simulink model "car_model"  (R2022b)
settings: Solver=VariableStepAuto  StartTime=0.0  StopTime=30  RelTol=1e-3
values from neighbouring files (symbols this model uses):
  X = Chassis_Signals.InertFrm.Cg.Disp.X.Data(:)    [Simulation_Data_Parse.m]    (also in Vehicle_Sim_Parse.m)
  Y = Chassis_Signals.InertFrm.Cg.Disp.Y.Data(:)    [Simulation_Data_Parse.m]    (also in Vehicle_Sim_Parse.m)
undefined symbols (not defined in the file or in its folder): ABS_MAX_TORQUE, ABS_MAX_TRQ_CMD, ABS_MIN_TORQUE, acc_IC, ACCELERATION_MAX, ActSuspDutyCycle, Aeq_left, Aeq_right, alpha_error, ang_acc_hystersesis, ang_IC, ang_vel_IC, area_air, axb, battery_current_IC, BATTERY_CURRENT_MAX, BATTERY_CURRENT_MIN, battery_FT_IC, battery_T_IC, BATTERY_TEMPERATURE_MAX, BATTERY_TEMPERATURE_MIN, battery_voltage_IC, BATTERY_VOLTAGE_MAX, BATTERY_VOLTAGE_MIN, Brake_Pressure_IC, ccl_IC, CENTER_STEER_ANGLE_MAX, covA, covarience_matrix_IC, covG, covM, covP, covV, cy_sweep, dB, dcl_IC, DCL_MAX, DCL_MIN, deadband_angle, dIndex, DiscIntNeverNeededParam, disk_abore, driver_t, dt_OFF, dt_ON, dTx, dx, dZ, F0z, forward_look_straight, forward_look_turn, fusion_t, fusion_t_sim, Fz_IC, Fz_sweep, g, gearbox_efficiency, gps_counter_IC, gps_ratio, gr ... (+105)
libraries: fl_lib x62, nesl_utility x16, vehdynlibtire x10, vehdynlibsuspension x8, simulink x5, autolibutils x5, sharedtransform x5, EngineCoolingComponents_lib x4, slpidlib x3, SimscapeFluids_lib x3, dspstat3 x2, shared6dof x2
(part 3 of 10)

== system car_model/Vehicle Model/Electronics/Cooling Sensors ==
  Analog Signals : Inport
  Bus Creator9 : BusCreator  Inputs=5
  Bus Selector : BusSelector  OutputSignals=trn.motor_temperature,trn.mc_temp,trn.motor_fluid_temperature,trn.battery_temperature,trn.battery_fluid_temperature
  Delay1 : Delay  InitialCondition=[1 1; 1 1; 1 1; 1 1].*motor_T_IC
  Delay11 : Delay  InitialCondition=[1 1; 1 1; 1 1; 1 1].*motor_T_IC
  Delay12 : Delay  InitialCondition=[1 1; 1 1].*motor_FT_IC
  Delay13 : Delay  InitialCondition=[1 1].*battery_T_IC
  Delay14 : Delay  InitialCondition=[1 1].*battery_FT_IC
  Rate Transition1 : RateTransition  InitialCondition=[1 1].*motor_FT_IC  OutPortSampleTime=0
  Rate Transition2 : RateTransition  OutPortSampleTime=0
  Rate Transition3 : RateTransition  OutPortSampleTime=0
  Saturation10 : Saturate  UpperLimit=MOTOR_TEMPERATURE_MAX  LowerLimit=MOTOR_TEMPERATURE_MIN
  Saturation11 : Saturate  UpperLimit=BATTERY_TEMPERATURE_MAX  LowerLimit=BATTERY_TEMPERATURE_MIN
  Saturation12 : Saturate  UpperLimit=BATTERY_TEMPERATURE_MAX  LowerLimit=BATTERY_TEMPERATURE_MIN
  Saturation18 : Saturate  UpperLimit=MOTOR_TEMPERATURE_MAX  LowerLimit=MOTOR_TEMPERATURE_MIN
  Saturation21 : Saturate  UpperLimit=MOTOR_TEMPERATURE_MAX  LowerLimit=MOTOR_TEMPERATURE_MIN
  Zero-Order Hold{1,11..14} (5 alike) : ZeroOrderHold  SampleTime=sensor_t
  Cooling Sensors : Outport
  wires:
  Delay1/1 -> Saturation21/1
  Saturation21/1 -> Bus Creator9/2  "mc_T"
  Bus Selector/2 -> Zero-Order Hold1/1  "<mc_temp>"
  Zero-Order Hold1/1 -> Delay1/1
  Delay14/1 -> Saturation12/1
  Delay11/1 -> Saturation18/1
  Delay12/1 -> Saturation10/1
  Saturation12/1 -> Bus Creator9/5  "batt_FT"
  Zero-Order Hold12/1 -> Delay12/1
  Zero-Order Hold14/1 -> Delay14/1
  Bus Selector/4 -> Rate Transition2/1  "<battery_temperature>"
  Zero-Order Hold11/1 -> Delay11/1
  Saturation18/1 -> Bus Creator9/1  "motor_T"
  Zero-Order Hold13/1 -> Delay13/1
  Bus Selector/3 -> Rate Transition1/1  "<motor_fluid_temperature>"
  Saturation11/1 -> Bus Creator9/4  "batt_T"
  Saturation10/1 -> Bus Creator9/3  "motor_FT"
  Delay13/1 -> Saturation11/1
  Bus Selector/1 -> Zero-Order Hold11/1  "<motor_temperature>"
  Bus Selector/5 -> Rate Transition3/1  "<battery_fluid_temperature>"
  Bus Creator9/1 -> Cooling Sensors/1
  Rate Transition1/1 -> Zero-Order Hold12/1  "motor_fluid_temperature"
  Rate Transition2/1 -> Zero-Order Hold13/1  "battery_temperature"
  Rate Transition3/1 -> Zero-Order Hold14/1  "battery_fluid_temperature"
  Analog Signals/1 -> Bus Selector/1

== system car_model/Vehicle Model/Electronics/Corner Dynamics Sensors ==
  Analog Signals : Inport
  Bus Creator10 : BusCreator  Inputs=4
  Bus Selector : BusSelector  OutputSignals=whl.TireFrame.Omega,sus.Sus.steering_angle,sus.Sus.shock_length,whl.TireFrame.GndFz
  Delay15 : Delay  InitialCondition=ones(1, 4, 2).*omega_IC
  Delay16 : Delay  InitialCondition=[1 1].*theta_IC
  Delay17 : Delay  InitialCondition=[1 1; 1 1; 1 1; 1 1].*shock_length_IC
  Delay18 : Delay  InitialCondition=[1 1; 1 1; 1 1; 1 1].*Fz_IC
  Saturation15 : Saturate  UpperLimit=SHOCK_LENGTH_MAX  LowerLimit=SHOCK_LENGTH_MIN
  Saturation16 : Saturate  UpperLimit=OMEGA_MAX  LowerLimit=OMEGA_MIN
  Saturation17 : Saturate  UpperLimit=1200  LowerLimit=200
  Saturation3 : Saturate  UpperLimit=CENTER_STEER_ANGLE_MAX  LowerLimit=-CENTER_STEER_ANGLE_MAX
  Transpose : Math  Operator=transpose
  Zero-Order Hold{15..18} (4 alike) : ZeroOrderHold  SampleTime=sensor_t
  Corner Dynamics Sensors : Outport
  wires:
  Transpose/1 -> Zero-Order Hold15/1  "omega"
  Bus Selector/1 -> Transpose/1  "<Omega>"
  Zero-Order Hold18/1 -> Delay18/1
  Delay18/1 -> Saturation17/1
  Zero-Order Hold15/1 -> Delay15/1
  Zero-Order Hold16/1 -> Delay16/1
  Saturation17/1 -> Bus Creator10/4  "FZ"
  Saturation3/1 -> Bus Creator10/2  "theta"
  Bus Selector/3 -> Zero-Order Hold17/1  "<shock_length>"
  Saturation15/1 -> Bus Creator10/3  "shock_L"
  Saturation16/1 -> Bus Creator10/1  "omega"
  Bus Selector/4 -> Zero-Order Hold18/1  "<GndFz>"
  Delay16/1 -> Saturation3/1
  Bus Selector/2 -> Zero-Order Hold16/1  "<steering_angle>"
  Delay17/1 -> Saturation15/1
  Delay15/1 -> Saturation16/1
  Zero-Order Hold17/1 -> Delay17/1
  Bus Creator10/1 -> Corner Dynamics Sensors/1
  Analog Signals/1 -> Bus Selector/1

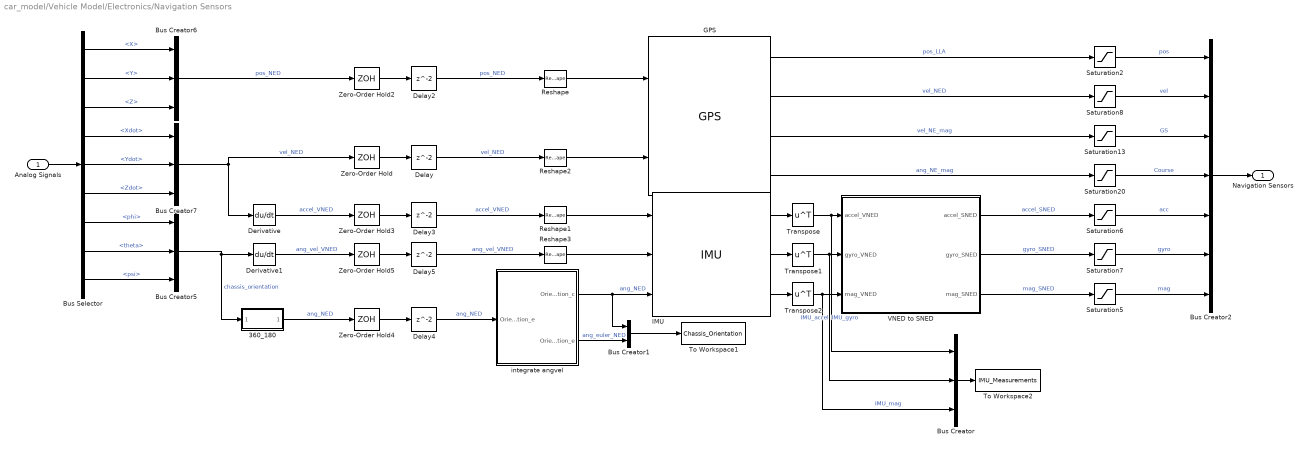
== system car_model/Vehicle Model/Electronics/Navigation Sensors ==
  Analog Signals : Inport
  360_180 : Subsystem
  Bus Creator : BusCreator  Inputs=IMU_accel,IMU_gyro,IMU_mag
  Bus Creator1 : BusCreator  Inputs=2
  Bus Creator2 : BusCreator  Inputs=7
  Bus Creator5 : BusCreator  Inputs=phi,theta,psi
  Bus Creator6 : BusCreator  Inputs=X,Y,Z
  Bus Creator7 : BusCreator  Inputs=Xdot,Ydot,Zdot
  Bus Selector : BusSelector  OutputSignals=veh.InertFrm.Cg.Disp.X,veh.InertFrm.Cg.Disp.Y,veh.InertFrm.Cg.Disp.Z,veh.InertFrm.Cg.Vel.Xdot,veh.InertFrm.Cg.Vel.Ydot,veh.InertFrm.Cg.Vel.Zdot,veh.InertFrm.Cg.Ang.phi,veh.InertFrm.Cg.Ang.theta,veh.InertFrm.Cg.Ang.psi
  Delay : Delay  InitialCondition=([1;1]*vel_IC)'
  Delay2 : Delay  InitialCondition=[1 1; 1 1; 1 1].*pos_IC
  Delay3 : Delay  InitialCondition=[1 1; 1 1; 1 1].*acc_IC
  Delay4 : Delay  InitialCondition=[1 1; 1 1; 1 1].*ang_IC
  Delay5 : Delay  InitialCondition=[1 1; 1 1; 1 1].*ang_vel_IC
  Derivative : Derivative
  Derivative1 : Derivative
  GPS : sensorgpslib/GPS  DispRefFrame=NED  PositionInputFormat=Local  ReferenceLocation=location_lla_IC  HorizontalPositionAccuracy=GPS_Z_ACCURACY  VerticalPositionAccuracy=GPS_XY_ACCURACY  VelocityAccuracy=GPS_V_ACCURACY  DecayFactor=GPS_NOISE_FACTOR  SeedDouble=r_GPS  SimulateUsing=Interpreted execution
      settings: LibrarySourceBlock=mspsensorlib/GPS
  IMU : mspsensorlib/IMU  DispRefFrame=NED  Temperature=25  MagneticFieldNED=mag_field_IC  MagneticFieldENU=[ -2.4169, 27.5550, 16.0849 ]  SeedDouble=r_IMU  SimulateUsing=Interpreted execution  AccelParamsMeasurementRange=ACC_MAX  AccelParamsResolution=ACC_RES  AccelParamsConstantBias=ACC_BIAS  AccelParamsAxesMisalignment=ACC_SKEW  AccelParamsNoiseDensity=ACC_VEL_WALK  AccelParamsBiasInstability=ACC_BIAS_INSTABILITY  AccelParamsRandomWalk=ACC_WALK  AccelParamsTemperatureBias=ACC_T_BIAS  AccelParamsTemperatureScaleFactor=ACC_T_SCALE  GyroParamsMeasurementRange=GYR_MAX  GyroParamsResolution=GYR_RES  GyroParamsConstantBias=GYR_BIAS  GyroParamsAxesMisalignment=GYR_SKEW  GyroParamsAccelerationBias=GYR_ACC_BIAS  GyroParamsNoiseDensity=GYR_ANG_WALK  GyroParamsBiasInstability=GYR_BIAS_INSTABILITY  GyroParamsRandomWalk=GYR_WALK  GyroParamsTemperatureBias=GYR_T_BIAS  GyroParamsTemperatureScaleFactor=GYR_T_SCALE  MagParamsMeasurementRange=MAG_MAX  MagParamsResolution=MAG_RES  MagParamsConstantBias=MAG_BIAS  MagParamsAxesMisalignment=MAG_SKEW  MagParamsNoiseDensity=MAG_WHITE  MagParamsBiasInstability=MAG_BIAS_INSTABILITY  MagParamsRandomWalk=MAG_WALK  MagParamsTemperatureBias=MAG_T_BIAS  MagParamsTemperatureScaleFactor=MAG_T_SCALE
  Reshape{,1..3} (4 alike) : Reshape  OutputDimensionality=Row vector (2-D)
  Saturation13 : Saturate  UpperLimit=VELOCITY_MAX  LowerLimit=-VELOCITY_MAX
  Saturation2 : Saturate  UpperLimit=inf  LowerLimit=-inf
  Saturation20 : Saturate  UpperLimit=ORIENTATION_MAX  LowerLimit=-ORIENTATION_MAX
  Saturation5 : Saturate  UpperLimit=MAG_MAX  LowerLimit=-MAG_MAX
  Saturation6 : Saturate  UpperLimit=ACCELERATION_MAX  LowerLimit=-ACCELERATION_MAX
  Saturation7 : Saturate  UpperLimit=YAW_MAX  LowerLimit=-YAW_MAX
  Saturation8 : Saturate  UpperLimit=VELOCITY_MAX  LowerLimit=-VELOCITY_MAX
  To Workspace1 : ToWorkspace  VariableName=Chassis_Orientation  SaveFormat=Timeseries  SampleTime=-1
  To Workspace2 : ToWorkspace  VariableName=IMU_Measurements  SaveFormat=Timeseries  SampleTime=-1
  Transpose : Math  Operator=transpose
  Transpose1 : Math  Operator=transpose
  Transpose2 : Math  Operator=transpose
  VNED to SNED : MATLAB Function  TreatAsAtomicUnit=on
  Zero-Order Hold{,2..5} (5 alike) : ZeroOrderHold  SampleTime=sensor_t
  integrate angvel : MATLAB Function  TreatAsAtomicUnit=on
  Navigation Sensors : Outport
  wires:
  Delay5/1 -> Reshape3/1  "ang_vel_VNED"
  Delay/1 -> Reshape2/1  "vel_NED"
  Delay3/1 -> Reshape1/1  "accel_VNED"
  Delay2/1 -> Reshape/1  "pos_NED"
  integrate angvel/1(Orientation_c) -> Bus Creator1/1, IMU/3  "ang_NED"
  GPS/4 -> Saturation20/1  "ang_NE_mag"
  GPS/3 -> Saturation13/1  "vel_NE_mag"
  GPS/2 -> Saturation8/1  "vel_NED"
  GPS/1 -> Saturation2/1  "pos_LLA"
  VNED to SNED/2(gyro_SNED) -> Saturation7/1  "gyro_SNED"
  VNED to SNED/1(accel_SNED) -> Saturation6/1  "accel_SNED"
  VNED to SNED/3(mag_SNED) -> Saturation5/1  "mag_SNED"
  Delay4/1 -> integrate angvel/1("Orientation_e ")  "ang_NED"
  Transpose2/1 -> Bus Creator/3, VNED to SNED/3(mag_VNED)  "IMU_mag"
  Transpose1/1 -> Bus Creator/2, VNED to SNED/2(gyro_VNED)  "IMU_gyro"
  Transpose/1 -> Bus Creator/1, VNED to SNED/1(accel_VNED)  "IMU_accel"
  IMU/3 -> Transpose2/1
  IMU/1 -> Transpose/1
  IMU/2 -> Transpose1/1
  Bus Creator/1 -> To Workspace2/1
  Bus Creator1/1 -> To Workspace1/1
  integrate angvel/2(Orientation_e) -> Bus Creator1/2  "ang_euler_NED"
  Zero-Order Hold/1 -> Delay/1
  Bus Creator7/1 -> Zero-Order Hold/1, Derivative/1  "vel_NED"
  Zero-Order Hold2/1 -> Delay2/1
  Bus Creator6/1 -> Zero-Order Hold2/1  "pos_NED"
  Zero-Order Hold3/1 -> Delay3/1
  Derivative/1 -> Zero-Order Hold3/1  "accel_VNED"
  Zero-Order Hold5/1 -> Delay5/1
  Derivative1/1 -> Zero-Order Hold5/1  "ang_vel_VNED"
  Zero-Order Hold4/1 -> Delay4/1
  360_180/1(psi_rev) -> Zero-Order Hold4/1  "ang_NED"
  Saturation2/1 -> Bus Creator2/1  "pos"
  Saturation13/1 -> Bus Creator2/3  "GS"
  Saturation6/1 -> Bus Creator2/5  "acc"
  Saturation20/1 -> Bus Creator2/4  "Course"
  Saturation5/1 -> Bus Creator2/7  "mag"
  Saturation8/1 -> Bus Creator2/2  "vel"
  Saturation7/1 -> Bus Creator2/6  "gyro"
  Bus Creator2/1 -> Navigation Sensors/1
  Bus Selector/1 -> Bus Creator6/1  "<X>"
  Bus Selector/8 -> Bus Creator5/2  "<theta>"
  Bus Selector/2 -> Bus Creator6/2  "<Y>"
  Bus Selector/6 -> Bus Creator7/3  "<Zdot>"
  Bus Selector/5 -> Bus Creator7/2  "<Ydot>"
  Bus Selector/4 -> Bus Creator7/1  "<Xdot>"
  Bus Selector/7 -> Bus Creator5/1  "<phi>"
  Bus Creator5/1 -> 360_180/1(<psi>), Derivative1/1  "chassis_orientation"
  Bus Selector/3 -> Bus Creator6/3  "<Z>"
  Bus Selector/9 -> Bus Creator5/3  "<psi>"
  Analog Signals/1 -> Bus Selector/1
  Reshape/1 -> GPS/1
  Reshape1/1 -> IMU/1
  Reshape2/1 -> GPS/2
  Reshape3/1 -> IMU/2

== system car_model/Vehicle Model/Electronics/Power Sensors ==
  Analog Signals : Inport
  Bus Creator8 : BusCreator  Inputs=5
  Bus Selector : BusSelector  OutputSignals=trn.battery_voltage,trn.battery_current,trn.motor_voltage,trn.motor_current,trn.power_limits
  Delay10 : Delay  InitialCondition=[dcl_IC; ccl_IC]*[1 1]
  Delay6 : Delay  InitialCondition=[1 1].*battery_voltage_IC
  Delay7 : Delay  InitialCondition=[1 1].*battery_current_IC
  Delay8 : Delay  InitialCondition=[1 1; 1 1; 1 1; 1 1].*motor_voltage_IC
  Delay9 : Delay  InitialCondition=ones(1, 4, 2).*motor_current_IC
  Saturation1 : Saturate  UpperLimit=BATTERY_CURRENT_MAX  LowerLimit=BATTERY_CURRENT_MIN
  Saturation14 : Saturate  UpperLimit=DCL_MAX  LowerLimit=DCL_MIN
  Saturation19 : Saturate  UpperLimit=BATTERY_VOLTAGE_MAX  LowerLimit=BATTERY_VOLTAGE_MIN
  Saturation4 : Saturate  UpperLimit=MOTOR_VOLTAGE_MAX  LowerLimit=MOTOR_VOLTAGE_MIN
  Saturation9 : Saturate  UpperLimit=MOTOR_CURRENT_MAX  LowerLimit=MOTOR_CURRENT_MIN
  Zero-Order Hold{6..10} (5 alike) : ZeroOrderHold  SampleTime=sensor_t
  Power Sensors : Outport
  wires:
  Zero-Order Hold6/1 -> Delay6/1
  Delay6/1 -> Saturation19/1
  Bus Selector/1 -> Zero-Order Hold6/1  "<battery_voltage>"
  Delay7/1 -> Saturation1/1
  Zero-Order Hold7/1 -> Delay7/1
  Bus Selector/2 -> Zero-Order Hold7/1  "<battery_current>"
  Delay8/1 -> Saturation4/1
  Zero-Order Hold8/1 -> Delay8/1
  Bus Selector/3 -> Zero-Order Hold8/1  "<motor_voltage>"
  Delay9/1 -> Saturation9/1
  Zero-Order Hold9/1 -> Delay9/1
  Bus Selector/4 -> Zero-Order Hold9/1  "<motor_current>"
  Zero-Order Hold10/1 -> Delay10/1
  Delay10/1 -> Saturation14/1
  Bus Selector/5 -> Zero-Order Hold10/1  "<power_limits>"
  Saturation19/1 -> Bus Creator8/1  "batt_V"
  Saturation1/1 -> Bus Creator8/2  "batt_I"
  Saturation9/1 -> Bus Creator8/4  "motor_I"
  Saturation4/1 -> Bus Creator8/3  "motor_V"
  Saturation14/1 -> Bus Creator8/5  "pwr_lmt"
  Bus Creator8/1 -> Power Sensors/1
  Analog Signals/1 -> Bus Selector/1

== system car_model/Vehicle Model/Powertrain/Battery Cooling Loop ==
  omega_m : Inport
  Battery_V : Inport  Port=2
  Battery_I : Inport  Port=3
  CL Battery Fans : Inport  Port=4
  CL Battery Pump : Inport  Port=5
  Vg : Inport  Port=6
  Battery Temperature : Outport
  Battery Fluid Temperature : Outport  Port=2

== system car_model/Vehicle Model/Powertrain/Drivetrain ==
  battery voltage : Inport
  throttle : Inport  Port=2
  motor speed : Inport  Port=3
  1-D Lookup Table : Lookup_n-D  NumberOfTableDimensions=1  LookupTableObject=''  BreakpointsForDimension1=speed_bp  BreakpointsForDimension1FirstPoint=10  BreakpointsForDimension2FirstPoint=10  BreakpointsForDimension1Spacing=12  BreakpointsForDimension2Spacing=12  BeginIndexSearchUsingPreviousIndexResult=on  Table=max_torque_table  ExtrapMethod=Clip  DiagnosticForOutOfRangeInput=Error  InternalRulePriority=Speed  RndMeth=Simplest
  1-D Lookup Table1 : Lookup_n-D  NumberOfTableDimensions=1  LookupTableObject=''  BreakpointsForDimension1=speed_bp  BreakpointsForDimension1FirstPoint=10  BreakpointsForDimension2FirstPoint=10  BreakpointsForDimension1Spacing=12  BreakpointsForDimension2Spacing=12  BeginIndexSearchUsingPreviousIndexResult=on  Table=max_current_table  ExtrapMethod=Clip  DiagnosticForOutOfRangeInput=Error  InternalRulePriority=Speed  RndMeth=Simplest
  Gain : Gain  Gain=MOTOR_ENABLE
  Gain1 : Gain  Gain=gr.*gearbox_efficiency
  Gain2 : Gain  Gain=MOTOR_ENABLE
  Mean : dspstat3/Mean  run=off  InputProcessing=Columns as channels (frame based)  reset_popup=None  directionMode=Entire input  dimension=1  roiEnable=off  roiType=Rectangles  roiPortion=Entire ROI  roiOutput=Individual statistics for each ROI  roiFlag=off  roundingMode=Floor  overflowMode=off  outputDataTypeStr=Inherit: Same as accumulator  outputMin=[]  outputMax=[]  outputLastDataTypeStr=Inherit: Same as accumulator
  Product : Product
  Product1 : Product
  Sum : Sum  Inputs=+
  Terminator : Terminator
  battery current : Outport
  wheel torque : Outport  Port=2
  motor torque : Outport  Port=3
  wires:
  1-D Lookup Table/1 -> Gain/1
  motor speed/1 -> 1-D Lookup Table1/1, Mean/1
  Product/1 -> motor torque/1, Gain1/1
  throttle/1 -> Product/1, Product1/1
  Gain/1 -> Product/2
  Gain1/1 -> wheel torque/1
  Sum/1 -> battery current/1
  battery voltage/1 -> Terminator/1
  Mean/1 -> 1-D Lookup Table/1
  1-D Lookup Table1/1 -> Gain2/1
  Gain2/1 -> Product1/2
  Product1/1 -> Sum/1
